simulink model "chap7_1sim"  (R2015a)
settings: Solver=ode45  StartTime=0.0  StopTime=10  FixedStep=0.01  RelTol=1e-3
settings Model: Creator=Masoud  LastModifiedBy=Masoud

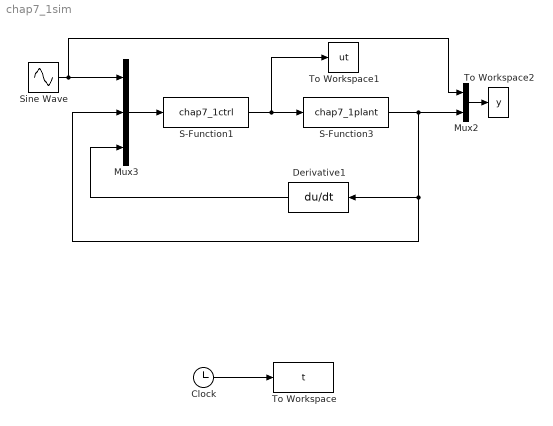
== system chap7_1sim ==
  Clock : Clock
  Derivative1 : Derivative
  Mux2 : Mux  Inputs=2
  Mux3 : Mux  Inputs=3
  S-Function1 : S-Function  FunctionName=chap7_1ctrl  SFunctionModules='chap7_1ctrl'
  S-Function3 : S-Function  FunctionName=chap7_1plant  SFunctionModules='chap7_1plant'
  Sine Wave : Sin  SampleTime=0
  To Workspace : ToWorkspace  VariableName=t  SampleTime=-1
  To Workspace1 : ToWorkspace  VariableName=ut  SampleTime=-1
  To Workspace2 : ToWorkspace  VariableName=y  SampleTime=-1
  wires:
  Clock/1 -> To Workspace/1
  Mux2/1 -> To Workspace2/1
  S-Function3/1 -> Mux3/2, Derivative1/1, Mux2/2
  S-Function1/1 -> S-Function3/1, To Workspace1/1
  Sine Wave/1 -> Mux3/1, Mux2/1
  Mux3/1 -> S-Function1/1
  Derivative1/1 -> Mux3/3
